simulink model "M_M_m_m"  (R2024b)
settings: Solver=VariableStepAuto  StartTime=0.0  StopTime=70000  RelTol=1e-3
values from neighbouring files (symbols this model uses):
  m = 1    [MMmKN_indicatori.m]    (also in MMmK_indicatori.m = 2; Perf_M_M_m.m = m(:)'; Perf_M_M_m_K.m = m(:)'; Perf_M_M_m_K_N.m = m(:)')
  R = Wq + r / mu    [Perf_M_Er_1.m]    (also in Perf_M_M_1.m = 1 ./ (mu .* (1 - rho)); Perf_M_M_1_K.m = Q ./ X; Perf_M_M_m.m = Q ./ lambda; Perf_M_M_m_K.m = zeros(size(lambda)))
undefined symbols (not defined in the file or in its folder): elapsedTime, entity, n
settings Model: Creator=atomu  LastModifiedBy=atomu

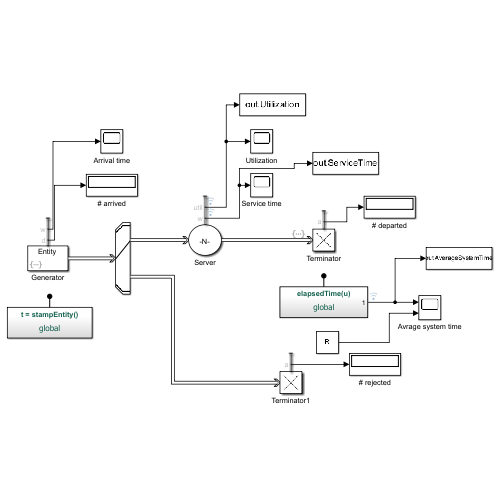
[thumbnail: Simulink's stored preview of the top-level diagram]
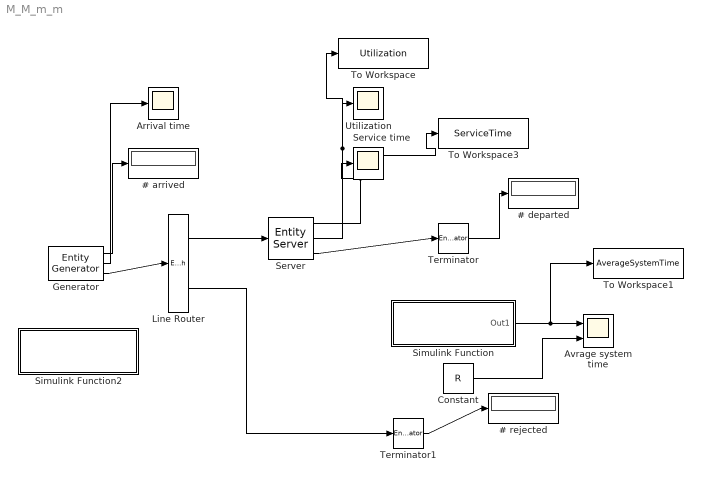
== system M_M_m_m ==
  # arrived : Display
  # departed : Display
  # rejected : Display
  Arrival time : Scope
  Avrage system time : Scope  NumInputPorts=2
  Constant : Constant  Value=R
  Generator : EntityGenerator  OutputPortMessageModes=n,n,m  TimeSource=MATLAB action  IntergenerationTimeAction=|  GenerateAction=|  AttributeName=TimeStamp  AttributeInitialValue=0  NumberEntitiesDeparted=on  AverageIntergenerationTime=on  EntityType=Structured  EntityTypeName=Entity
      IntergenerationTimeAction=|
      | persistent rngInit;
      | if isempty(rngInit)
      |     seed = 12345;
      |     rng(seed);
      |     rngInit = true;
      | end
      | 
      | % Pattern: Exponential distribution
      | med = 1/lambda;
      | dt = -med * log(1 - rand());
      GenerateAction=|
      | % Record time of generation so we can
      | % compute system time
      | entity.TimeStamp = stampEntity();
      settings: OutputPortMap=o0,o2,o3
  Line Router : EntityOutputSwitch  InputPortMessageModes=m  OutputPortMessageModes=m,m  SwitchAttributeName=QueuePath
  Server : EntityServer  InputPortMessageModes=m  OutputPortMessageModes=n,n,m  Capacity=ServerNumbers  ServiceTimeSource=MATLAB action  ServiceTimeAction=|  AverageWait=on  Utilization=on
      | persistent rngInit;
      | if isempty(rngInit)
      |     seed = 25487;
      |     rng(seed);
      |     rngInit = true;
      | end
      | 
      | % Pattern: Exponential distribution
      | med= 1/mu;
      | dt = -med * log(1 - rand());
      settings: OutputPortMap=o4,o5,o9
  Service time : Scope
  Simulink Function : Subsystem  TreatAsAtomicUnit=on
  Simulink Function2 : Subsystem  TreatAsAtomicUnit=on
  Terminator : EntityTerminator  InputPortMessageModes=m  EntryAction=elapsedTime(entity.TimeStamp)  NumberEntitiesArrived=on
      settings: OutputPortMap=o0
  Terminator1 : EntityTerminator  InputPortMessageModes=m  NumberEntitiesArrived=on
      settings: OutputPortMap=o0
  To Workspace : ToWorkspace  VariableName=Utilization  SaveFormat=Timeseries  SampleTime=-1
  To Workspace1 : ToWorkspace  VariableName=AverageSystemTime  SaveFormat=Timeseries  SampleTime=-1
  To Workspace3 : ToWorkspace  VariableName=ServiceTime  SaveFormat=Timeseries  SampleTime=-1
  Utilization : Scope
  wires:
  Constant/1 -> Avrage system time/2
  Server/2 -> To Workspace/1, Utilization/1
  Server/3 -> Terminator/1
  Generator/1 -> # arrived/1
  Generator/2 -> Arrival time/1
  Server/1 -> To Workspace3/1, Service time/1
  Terminator/1 -> # departed/1
  Simulink Function/1(Out1) -> To Workspace1/1, Avrage system time/1
  Line Router/1 -> Server/1
  Generator/3 -> Line Router/1
  Line Router/2 -> Terminator1/1
  Terminator1/1 -> # rejected/1

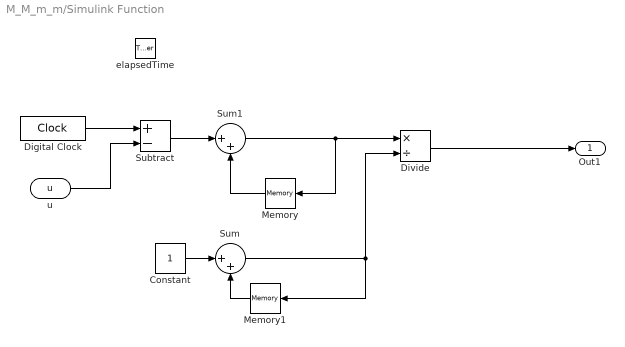
== system M_M_m_m/Simulink Function ==
  elapsedTime : TriggerPort  TriggerType=function-call  IsSimulinkFunction=on  FunctionName=elapsedTime  VariantControl=Variant
  Constant : Constant
  Digital Clock : DigitalClock  SampleTime=-1
  Divide : Product  Inputs=*/
  Memory : Memory  InheritSampleTime=on
  Memory1 : Memory  InheritSampleTime=on
  Subtract : Sum  Inputs=+-
  Sum : Sum  Inputs=|++
  Sum1 : Sum  Inputs=|++
  u : ArgIn  DisableCoverage=on  ArgumentName=u
  Out1 : Outport
  wires:
  Digital Clock/1 -> Subtract/1
  u/1 -> Subtract/2
  Subtract/1 -> Sum1/1
  Constant/1 -> Sum/1
  Memory1/1 -> Sum/2
  Sum/1 -> Memory1/1, Divide/2
  Divide/1 -> Out1/1
  Sum1/1 -> Memory/1, Divide/1
  Memory/1 -> Sum1/2

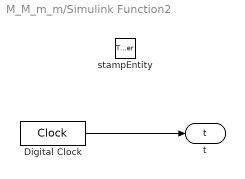
== system M_M_m_m/Simulink Function2 ==
  stampEntity : TriggerPort  TriggerType=function-call  IsSimulinkFunction=on  FunctionName=stampEntity  VariantControl=Variant
  Digital Clock : DigitalClock  SampleTime=-1
  t : ArgOut  DisableCoverage=on  ArgumentName=t
  wires:
  Digital Clock/1 -> t/1
